simulink model "PLC_reg_na_C"  (R2021b)
settings: Solver=ode14x  StartTime=0.0  StopTime=10.0  FixedStep=0.2  RelTol=1e-3
libraries: slpidlib x1
settings Model: Creator=Alex  LastModifiedBy=79159
settings SolverCC: AlgebraicLoopSolver=TrustRegion
settings DataIOCC: ReturnWorkspaceOutputs=off
settings DebuggingCC: SFMachineParentedDataDiag=warning  ArithmeticOperatorsInVariantConditions=warning
settings SFSimCC: SimUseLocalCustomCode=off  CustomCodeUndefinedFunction=UseInterfaceOnly
settings RTWCC: RTWUseLocalCustomCode=off

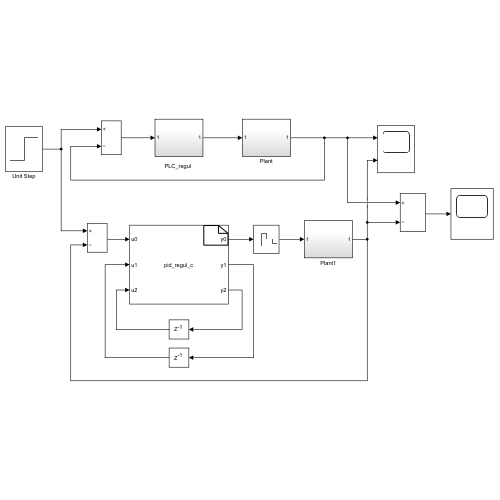
[thumbnail: Simulink's stored preview of the top-level diagram]
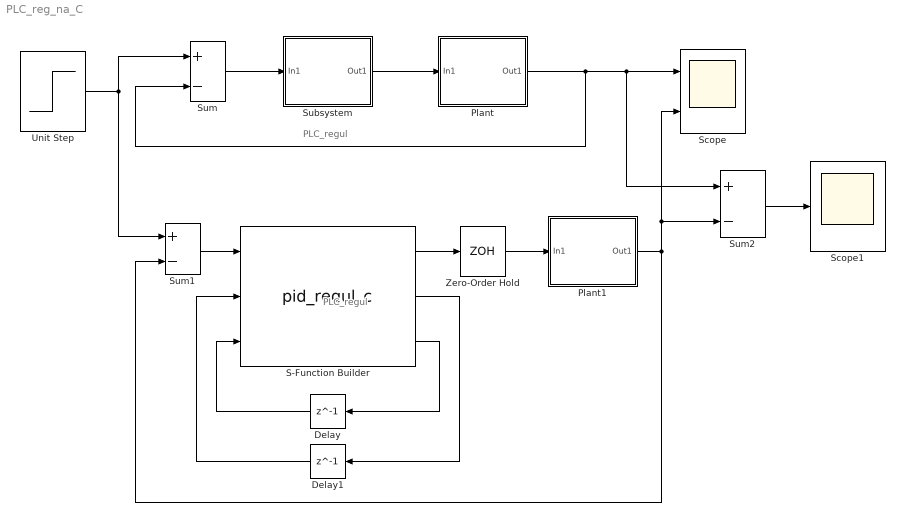
== system PLC_reg_na_C ==
  note: PLC_regul
  note: PLC_regul
  Delay : Delay  DelayLength=1
  Delay1 : Delay  DelayLength=1
  Plant : Subsystem
  Plant1 : Subsystem
  S-Function Builder : S-Function  InitFcn=try, set_param(gcb,'FunctionName','pid_regul_c'), end  FunctionName=pid_regul_c  SFunctionModules=pid_regul_c_wrapper  SFunctionDeploymentMode=off  EnableBusSupport=off  mask(S-Function Builder){}
      mask help: Simulink:masks:SFunctionBuilder_MD
      mask init:
      | val = [[.9  0.75 0.75 1 1 .9 .9 1]',[1 1 0.75 0.75 .9 .9 1 .9]'];try , sys = get_param(gcb,'SfunBuilderFcnName');if isempty(sys), sys = get_param(gcb,'FunctionName'); end,catch, sys = get_param(gcb,'FunctionName'); end
      settings: CopyFcn=set_param(gcbh,'LinkStatus','none')  PreSaveFcn=try, set_param(gcb,'FunctionName','pid_regul_c'), end  OpenFcn=sfunctionwizard(gcbh)
      mask Display: plot(val(:,1),val(:,2)),disp(sys),port_label('input',1,'u0'),port_label('input',2,'u1'),port_label('input',3,'u2'),port_label('output',1,'y0'),port_label('output',2,'y1'),port_label('output',3,'y2')
  Scope : Scope  NumInputPorts=2
  Scope1 : Scope
  Subsystem : Subsystem
  Sum : Sum  Inputs=+-  InputSameDT=on  SaturateOnIntegerOverflow=on  OutDataTypeStr=Inherit: Same as first input
  Sum1 : Sum  Inputs=+-  InputSameDT=on  SaturateOnIntegerOverflow=on  OutDataTypeStr=Inherit: Same as first input
  Sum2 : Sum  Inputs=+-  InputSameDT=on  SaturateOnIntegerOverflow=on  OutDataTypeStr=Inherit: Same as first input
  Unit Step : Step  Time=0  SampleTime=0
  Zero-Order Hold : ZeroOrderHold  SampleTime=0.2
  wires:
  Plant/1(Out1) -> Sum/2, Sum2/1, Scope/1
  Unit Step/1 -> Sum1/1, Sum/1
  Sum/1 -> Subsystem/1(In1)
  Subsystem/1(Out1) -> Plant/1(In1)
  Plant1/1(Out1) -> Sum1/2, Scope/2, Sum2/2
  Sum1/1 -> S-Function Builder/1
  S-Function Builder/3 -> Delay/1
  Delay/1 -> S-Function Builder/3
  S-Function Builder/2 -> Delay1/1
  Delay1/1 -> S-Function Builder/2
  S-Function Builder/1 -> Zero-Order Hold/1
  Zero-Order Hold/1 -> Plant1/1(In1)
  Sum2/1 -> Scope1/1

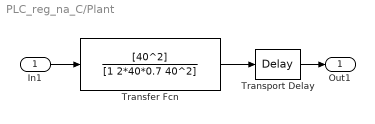
== system PLC_reg_na_C/Plant ==
  In1 : Inport
  Transfer Fcn : TransferFcn  Numerator=[40^2]  Denominator=[1 2*40*0.7 40^2]
  Transport Delay : TransportDelay
  Out1 : Outport  VectorParamsAs1DForOutWhenUnconnected=off
  wires:
  Transfer Fcn/1 -> Transport Delay/1
  In1/1 -> Transfer Fcn/1
  Transport Delay/1 -> Out1/1

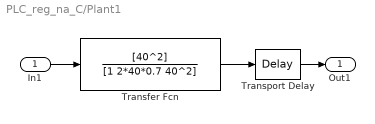
== system PLC_reg_na_C/Plant1 ==
  In1 : Inport
  Transfer Fcn : TransferFcn  Numerator=[40^2]  Denominator=[1 2*40*0.7 40^2]
  Transport Delay : TransportDelay
  Out1 : Outport  VectorParamsAs1DForOutWhenUnconnected=off
  wires:
  Transfer Fcn/1 -> Transport Delay/1
  In1/1 -> Transfer Fcn/1
  Transport Delay/1 -> Out1/1

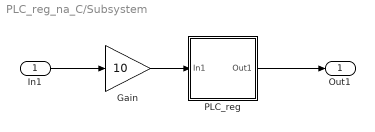
== system PLC_reg_na_C/Subsystem ==
  In1 : Inport
  Gain : Gain  Gain=10
  PLC_reg : Subsystem
  Out1 : Outport  VectorParamsAs1DForOutWhenUnconnected=off
  wires:
  Gain/1 -> PLC_reg/1(In1)
  In1/1 -> Gain/1
  PLC_reg/1(Out1) -> Out1/1

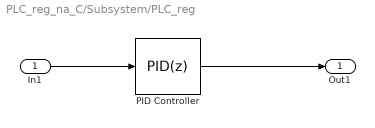
== system PLC_reg_na_C/Subsystem/PLC_reg ==
  In1 : Inport
  PID Controller : slpidlib/PID Controller  Controller=PID  Form=Parallel  TimeDomain=Discrete-time  UseExternalTs=off  SampleTime=0.2  IntegratorMethod=Forward Euler  FilterMethod=Forward Euler  ControllerParametersSource=internal  P=0.004333  I=0.04333  D=0  UseFilter=on  N=100  TunerSelectOption=Transfer Function Based (PID Tuner App)  InitialConditionSource=internal  InitialConditionForIntegrator=0  InitialConditionForFilter=0  DifferentiatorICPrevScaledInput=0  ExternalReset=none  TrackingMode=off  Kt=1  LimitOutput=off  SatLimitsSource=internal  UpperSaturationLimit=inf  LowerSaturationLimit=-inf  LinearizeAsGain=off  AntiWindupMode=none  Kb=1  POutMin=[]  POutMax=[]  IOutMin=[]  IOutMax=[]  DOutMin=[]  DOutMax=[]  NOutMin=[]  NOutMax=[]  SumOutMin=[]  SumOutMax=[]  SaturationOutMin=[]  SaturationOutMax=[]  PParamMin=[]  PParamMax=[]  IParamMin=[]  IParamMax=[]  DParamMin=[]  DParamMax=[]  NParamMin=[]  NParamMax=[]  KbParamMin=[]  KbParamMax=[]  KtParamMin=[]  KtParamMax=[]  KbOutMin=[]  KbOutMax=[]  KtOutMin=[]  KtOutMax=[]  IntegratorOutMin=[]  IntegratorOutMax=[]  FilterOutMin=[]  FilterOutMax=[]  SumI1OutMin=[]  SumI1OutMax=[]  SumI2OutMin=[]  SumI2OutMax=[]  SumI3OutMin=[]  SumI3OutMax=[]  SumI4OutMin=[]  SumI4OutMax=[]  SumDOutMin=[]  SumDOutMax=[]  DifferentiatorOutMin=[]  DifferentiatorOutMax=[]  FilterDiffOutCoefMin=[]  FilterDiffOutCoefMax=[]  ReciprocalOutMin=[]  ReciprocalOutMax=[]  SumDenOutMin=[]  SumDenOutMax=[]  SumNumOutMin=[]  SumNumOutMax=[]  DivideOutMin=[]  DivideOutMax=[]  UdiffTsProdOutMin=[]  UdiffTsProdOutMax=[]  NTsProdOutMin=[]  NTsProdOutMax=[]  UintegralTsProdOutMin=[]  UintegralTsProdOutMax=[]  UngainTsProdOutMin=[]  UngainTsProdOutMax=[]  IntegratorContinuousStateAttributes=''  IntegratorStateMustResolveToSignalObject=off  IntegratorRTWStateStorageClass=Auto  FilterContinuousStateAttributes=''  FilterStateMustResolveToSignalObject=off  FilterRTWStateStorageClass=Auto  ParallelPVariant=InternalParameters  IdealPVariant=Disabled  IVariant=InternalParameters  DVariant=InternalParameters  IntegratorVariant=Discrete  SatVariant=Disabled  AWVariant=Passthrough  PCopyVariant=Disabled  TRVariant=Disabled  FdbkBlocksVariant=Forward  IdealPFdbkVariant=Disabled  SatFdbkVariant=Disabled  DerivativeFilterVariant=ForwardEulerFilter  NVariant=InternalParameters  NCopyVariant=Disabled  FilterICVariant=InternalICsFilter  IntegratorICVariant=InternalICs  ExternalResetVariant=Disabled  TRSumVariant=Passthrough  SumFdbkVariant=Disabled  SumVariant=Sum_PID  TsampFilterVariant=InternalTs  TsampNgainVariant=Passthrough  TsampIntegralVariant=Passthrough  ExternalSaturationOutDataTypeStr=Inherit: Same as second input
  Out1 : Outport  VectorParamsAs1DForOutWhenUnconnected=off
  wires:
  In1/1 -> PID Controller/1
  PID Controller/1 -> Out1/1
